simulink model "sampleModel175"  (R2021b)
settings: Solver=VariableStepAuto  StartTime=0.0  StopTime=10.0  RelTol=1e-3
libraries: simulink x10
settings Model: Creator=user  LastModifiedBy=user

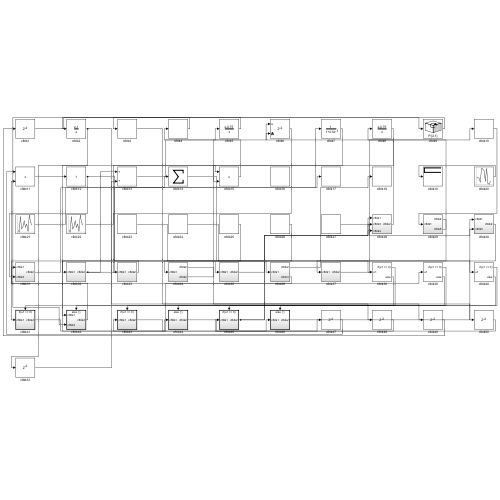
[thumbnail: Simulink's stored preview of the top-level diagram]
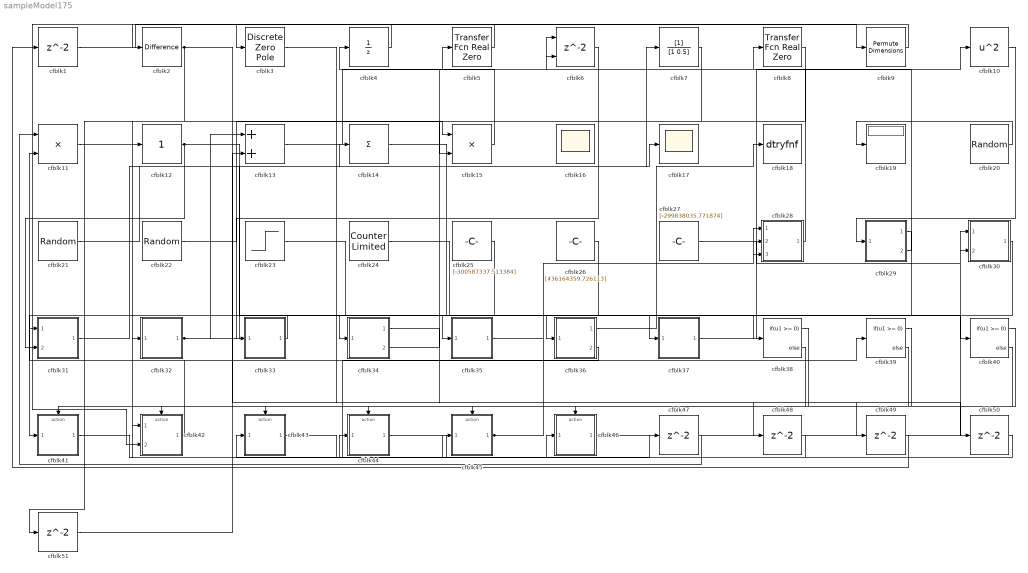
== system sampleModel175 ==
  cfblk{1,47..51} (6 alike) : Delay  SampleTime=1
  cfblk10 : Math  Operator=square  SaturateOnIntegerOverflow=on
  cfblk11 : Product  Inputs=**
  cfblk12 : simulink/Math Operations/Slider Gain  gain=1  low=0  high=2
  cfblk13 : Sum
  cfblk14 : Sum  Inputs=+
  cfblk15 : Product  Inputs=**
  cfblk16 : Scope
      settings: Floating=on
  cfblk17 : Scope
  cfblk18 : ToWorkspace  VariableName=dtryfnf  SaveFormat=Timeseries  SampleTime=-1
  cfblk19 : Display
  cfblk2 : simulink/Discrete/Difference  ICPrevInput=0.0  OutMin=[]  OutMax=[]  OutDataTypeStr=Inherit: Inherit via back propagation  OutDataType=fixdt(1, 16)  OutScaling=2^-10  DoSatur=off
  cfblk20 : RandomNumber  Mean=[-86357.100139]  Variance=[81821.434767]  Seed=[451125868.000000]  SampleTime=0.1
  cfblk21 : UniformRandomNumber  Minimum=[-1874443180.751388]  Maximum=[4408331130.961056]  Seed=[33260809.000000]  SampleTime=0.1
  cfblk22 : UniformRandomNumber  Minimum=[-459376011.363916]  Maximum=[9712076269.160019]  Seed=[42095909.000000]  SampleTime=0.1
  cfblk23 : Step  Time=[49.000000]  Before=[-237098877.927224]  After=[732105362.691046]  SampleTime=0
  cfblk24 : simulink/Sources/Counter Limited  uplimit=[157.000000]  tsamp=-1
  cfblk25 : Constant  Value=[-300587337.513384]  SampleTime=1
  cfblk26 : Constant  Value=[436164359.726113]  SampleTime=1
  cfblk27 : Constant  Value=[-299838035.771874]  SampleTime=1
  cfblk28 : Subsystem
  cfblk29 : Subsystem
  cfblk3 : DiscreteZeroPole  Poles=[0 0.5]  Gain=1
  cfblk30 : Subsystem
  cfblk31 : Subsystem
  cfblk32 : Subsystem
  cfblk33 : Subsystem
  cfblk34 : Subsystem
  cfblk35 : Subsystem
  cfblk36 : Subsystem
  cfblk37 : Subsystem
  cfblk38 : If  IfExpression=u1 >= 0  SampleTime=1
  cfblk39 : If  IfExpression=u1 >= 0  SampleTime=1
  cfblk4 : UnitDelay  HasFrameUpgradeWarning=on
  cfblk40 : If  IfExpression=u1 >= 0  SampleTime=1
  cfblk41 : Subsystem  TreatAsAtomicUnit=on
  cfblk42 : Subsystem  TreatAsAtomicUnit=on
  cfblk43 : Subsystem  TreatAsAtomicUnit=on
  cfblk44 : Subsystem  TreatAsAtomicUnit=on
  cfblk45 : Subsystem  TreatAsAtomicUnit=on
  cfblk46 : Subsystem  TreatAsAtomicUnit=on
  cfblk5 : simulink/Discrete/Transfer Fcn Real Zero  ZeroZ=0.75  ICPrevInput=0.0  DoSatur=off
      settings: SourceProductBaseCode=SL
  cfblk6 : Delay  ShowEnablePort=on  SampleTime=1
      settings: InputPortMap=u0,e6
  cfblk7 : DiscreteFilter  SampleTime=1
  cfblk8 : simulink/Discrete/Transfer Fcn Real Zero  ZeroZ=0.75  ICPrevInput=0.0  DoSatur=off
      settings: SourceProductBaseCode=SL
  cfblk9 : PermuteDimensions
  wires:
  cfblk32/1(cfblk2) -> cfblk17/1, cfblk13/1
  cfblk2/1 -> cfblk50/1, cfblk51/1
  cfblk44/1(cfblk2) -> cfblk46/1(cfblk1)
  cfblk29/1(cfblk2) -> cfblk34/1(cfblk1)
  cfblk46/1(cfblk2) -> cfblk30/1(cfblk1)
  cfblk11/1 -> cfblk39/1
  cfblk37/1(cfblk2) -> cfblk10/1
  cfblk20/1 -> cfblk19/1
  cfblk27/1 -> cfblk30/2(cfblk3)
  cfblk22/1 -> cfblk15/1
  cfblk25/1 -> cfblk42/1(cfblk1)
  cfblk10/1 -> cfblk29/1(cfblk1)
  cfblk13/1 -> cfblk5/1
  cfblk33/1(cfblk2) -> cfblk32/1(cfblk1)
  cfblk9/1 -> cfblk42/2(cfblk3)
  cfblk26/1 -> cfblk41/1(cfblk1)
  cfblk4/1 -> cfblk3/1
  cfblk36/1(cfblk2) -> cfblk18/1
  cfblk30/1(cfblk2) -> cfblk37/1(cfblk1)
  cfblk21/1 -> cfblk7/1
  cfblk23/1 -> cfblk35/1(cfblk1)
  cfblk1/1 -> cfblk9/1
  cfblk24/1 -> cfblk36/1(cfblk1)
  cfblk6/1 -> cfblk33/1(cfblk1)
  cfblk7/1 -> cfblk12/1
  cfblk14/1 -> cfblk38/1
  cfblk8/1 -> cfblk15/2
  cfblk34/2(cfblk4) -> cfblk6/1
  cfblk5/1 -> cfblk2/1
  cfblk41/1(cfblk2) -> cfblk44/1(cfblk1)
  cfblk42/1(cfblk2) -> cfblk11/2
  cfblk36/2(cfblk3) -> cfblk31/1(cfblk1)
  cfblk45/1(cfblk2) -> cfblk28/1(cfblk1), cfblk28/3(cfblk4)
  cfblk28/1(cfblk2) -> cfblk8/1
  cfblk29/2(cfblk5) -> cfblk6/2
  cfblk12/1 -> cfblk31/2(cfblk3), cfblk40/1
  cfblk35/1(cfblk2) -> cfblk28/2(cfblk3)
  cfblk15/1 -> cfblk4/1
  cfblk31/1(cfblk2) -> cfblk14/1
  cfblk38/1 -> cfblk41/Action
  cfblk38/2 -> cfblk42/Action
  cfblk39/1 -> cfblk43/Action
  cfblk39/2 -> cfblk44/Action
  cfblk40/1 -> cfblk45/Action
  cfblk40/2 -> cfblk46/Action
  cfblk43/1(cfblk2) -> cfblk47/1
  cfblk47/1 -> cfblk11/1
  cfblk34/1(cfblk2) -> cfblk48/1
  cfblk48/1 -> cfblk45/1(cfblk1)
  cfblk3/1 -> cfblk49/1
  cfblk49/1 -> cfblk1/1
  cfblk50/1 -> cfblk43/1(cfblk1)
  cfblk51/1 -> cfblk13/2

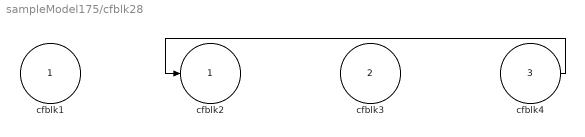
== system sampleModel175/cfblk28 ==
  cfblk1 : Inport
  cfblk3 : Inport  Port=2
  cfblk4 : Inport  Port=3
  cfblk2 : Outport
  wires:
  cfblk4/1 -> cfblk2/1

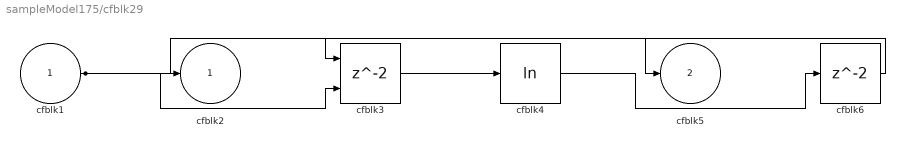
== system sampleModel175/cfblk29 ==
  cfblk1 : Inport
  cfblk3 : Delay  ShowEnablePort=on  SampleTime=1
      settings: InputPortMap=u0,e6
  cfblk4 : Math  Operator=log  SaturateOnIntegerOverflow=on
  cfblk6 : Delay  SampleTime=1
  cfblk2 : Outport
  cfblk5 : Outport  Port=2
  wires:
  cfblk1/1 -> cfblk5/1, cfblk2/1, cfblk3/2
  cfblk3/1 -> cfblk4/1
  cfblk4/1 -> cfblk6/1
  cfblk6/1 -> cfblk3/1

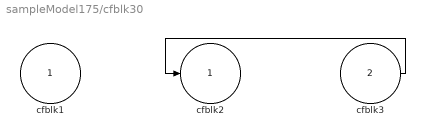
== system sampleModel175/cfblk30 ==
  cfblk1 : Inport
  cfblk3 : Inport  Port=2
  cfblk2 : Outport
  wires:
  cfblk3/1 -> cfblk2/1

== system sampleModel175/cfblk31 ==
  cfblk1 : Inport
  cfblk3 : Inport  Port=2
  cfblk2 : Outport
  wires:
  cfblk1/1 -> cfblk2/1

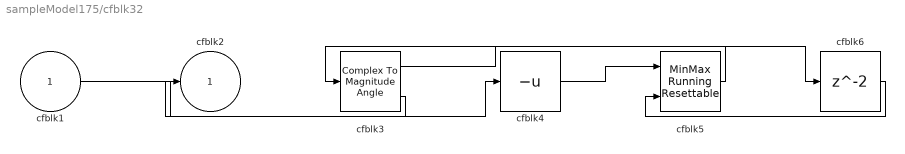
== system sampleModel175/cfblk32 ==
  cfblk1 : Inport
  cfblk3 : ComplexToMagnitudeAngle
  cfblk4 : UnaryMinus
  cfblk5 : simulink/Math Operations/MinMax Running Resettable  Function=min  vinit=0.0
  cfblk6 : Delay  SampleTime=1
  cfblk2 : Outport
  wires:
  cfblk4/1 -> cfblk5/1
  cfblk1/1 -> cfblk4/1
  cfblk5/1 -> cfblk3/1
  cfblk3/2 -> cfblk2/1
  cfblk3/1 -> cfblk6/1
  cfblk6/1 -> cfblk5/2

== system sampleModel175/cfblk33 ==
  cfblk1 : Inport
  cfblk3 : simulink/Math Operations/Slider Gain  gain=1  low=0  high=2
  cfblk2 : Outport
  wires:
  cfblk3/1 -> cfblk2/1
  cfblk1/1 -> cfblk3/1

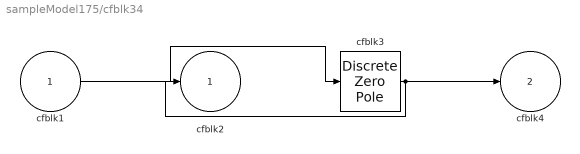
== system sampleModel175/cfblk34 ==
  cfblk1 : Inport
  cfblk3 : DiscreteZeroPole  Poles=[0 0.5]  Gain=1
  cfblk2 : Outport
  cfblk4 : Outport  Port=2
  wires:
  cfblk1/1 -> cfblk3/1
  cfblk3/1 -> cfblk2/1, cfblk4/1

== system sampleModel175/cfblk35 ==
  cfblk1 : Inport
  cfblk3 : Constant  Value=[711478801.923983]  SampleTime=1
  cfblk2 : Outport
  wires:
  cfblk3/1 -> cfblk2/1

== system sampleModel175/cfblk36 ==
  cfblk1 : Inport
  cfblk2 : Outport
  cfblk3 : Outport  Port=2
  wires:
  cfblk1/1 -> cfblk2/1, cfblk3/1

== system sampleModel175/cfblk37 ==
  cfblk1 : Inport
  cfblk3 : Delay  SampleTime=1
  cfblk2 : Outport
  wires:
  cfblk1/1 -> cfblk2/1, cfblk3/1

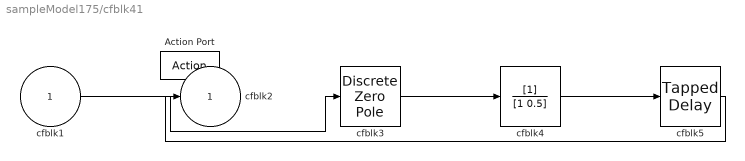
== system sampleModel175/cfblk41 ==
  cfblk1 : Inport
  Action Port : ActionPort  ActionPortLabel=if(u1 >= 0)
  cfblk3 : DiscreteZeroPole  Poles=[0 0.5]  Gain=1  SampleTime=-1
  cfblk4 : DiscreteFilter
  cfblk5 : simulink/Discrete/Tapped Delay  vinit=0.0  samptime=-1  NumDelays=1  DelayOrder=Oldest  includeCurrent=off
  cfblk2 : Outport
  wires:
  cfblk1/1 -> cfblk3/1
  cfblk5/1 -> cfblk2/1
  cfblk3/1 -> cfblk4/1
  cfblk4/1 -> cfblk5/1

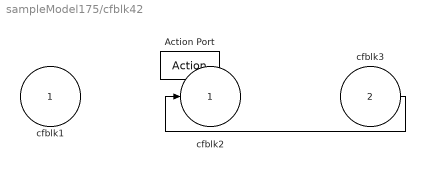
== system sampleModel175/cfblk42 ==
  cfblk1 : Inport
  cfblk3 : Inport  Port=2
  Action Port : ActionPort  ActionPortLabel=else
  cfblk2 : Outport
  wires:
  cfblk3/1 -> cfblk2/1

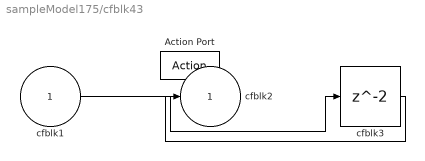
== system sampleModel175/cfblk43 ==
  cfblk1 : Inport
  Action Port : ActionPort  ActionPortLabel=if(u1 >= 0)
  cfblk3 : Delay
  cfblk2 : Outport
  wires:
  cfblk1/1 -> cfblk3/1
  cfblk3/1 -> cfblk2/1

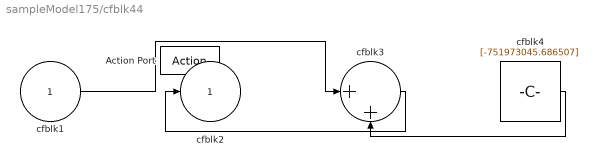
== system sampleModel175/cfblk44 ==
  cfblk1 : Inport
  Action Port : ActionPort  ActionPortLabel=else
  cfblk3 : Sum  Inputs=|++
  cfblk4 : Constant  Value=[-751973045.686507]  SampleTime=1
  cfblk2 : Outport
  wires:
  cfblk3/1 -> cfblk2/1
  cfblk1/1 -> cfblk3/1
  cfblk4/1 -> cfblk3/2

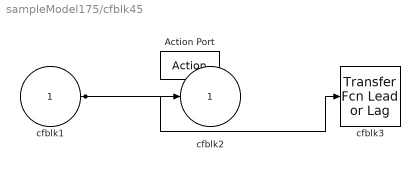
== system sampleModel175/cfblk45 ==
  cfblk1 : Inport
  Action Port : ActionPort  ActionPortLabel=if(u1 >= 0)
  cfblk3 : simulink/Discrete/Transfer Fcn Lead or Lag  PoleZ=0.95  ZeroZ=0.75  ICPrevOutput=0.0  ICPrevInput=0.0  DoSatur=off
      settings: SourceProductBaseCode=SL
  cfblk2 : Outport
  wires:
  cfblk1/1 -> cfblk2/1, cfblk3/1

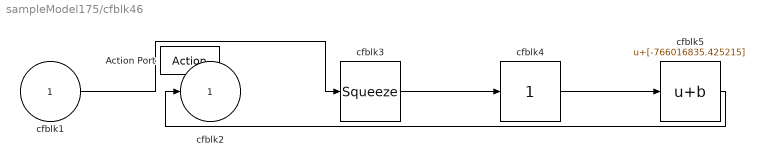
== system sampleModel175/cfblk46 ==
  cfblk1 : Inport
  Action Port : ActionPort  ActionPortLabel=else
  cfblk3 : Squeeze
  cfblk4 : simulink/Math Operations/Slider Gain  gain=1  low=0  high=2
  cfblk5 : Bias  Bias=[-766016835.425215]
  cfblk2 : Outport
  wires:
  cfblk4/1 -> cfblk5/1
  cfblk3/1 -> cfblk4/1
  cfblk5/1 -> cfblk2/1
  cfblk1/1 -> cfblk3/1
